simulink model "SSSC"  (R2022b)
settings: Solver=VariableStepAuto  StartTime=0.0  StopTime=.1  RelTol=1e-3
libraries: dspsigops x4, spsSeriesRLCBranchLib x3, simulink x2, spsDCVoltageSourceLib x2, spsMosfetLib x2, spsVoltageMeasurementLib x2, spsACVoltageSourceLib x1, spsCurrentMeasurementLib x1, spsTriangleGeneratorLib x1, sps_lib x1
settings Model: Creator=HP  LastModifiedBy=rishi kumar singh

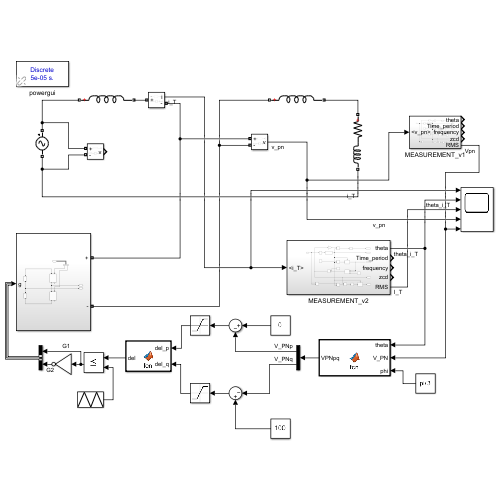
[thumbnail: Simulink's stored preview of the top-level diagram]
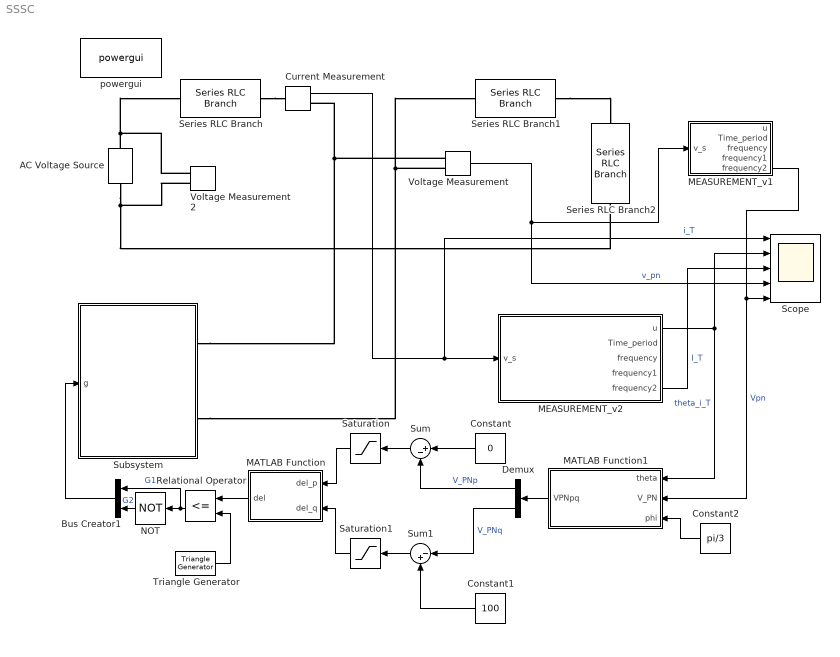
== system SSSC ==
  AC Voltage Source : spsACVoltageSourceLib/AC Voltage Source  Amplitude=20e3*sqrt(2)  Phase=0  Frequency=50  SampleTime=0  Measurements=None  BusType=swing  Pref=10e3  Qref=0  Qmin=-inf  Qmax=+inf
  Bus Creator1 : BusCreator  Inputs=2
  Constant : Constant  Value=0
  Constant1 : Constant  Value=100
  Constant2 : Constant  Value=pi/3
  Current Measurement : spsCurrentMeasurementLib/Current Measurement  PhasorSimulation=off  OutputType=Complex  PSBequivalent=0
  Demux : Demux  Outputs=2
  MATLAB Function : MATLAB Function  TreatAsAtomicUnit=on
  MATLAB Function1 : MATLAB Function  TreatAsAtomicUnit=on
  MEASUREMENT_v1 : Subsystem
  MEASUREMENT_v2 : Subsystem
  NOT : Logic  Operator=NOT  IconShape=distinctive  AllPortsSameDT=off  OutDataTypeStr=boolean
  Relational Operator : RelationalOperator  Operator=<=  OutDataTypeStr=boolean  RndMeth=Simplest  InputSameDT=off
  Saturation : Saturate
  Saturation1 : Saturate
  Scope : Scope  NumInputPorts=5
  Series RLC Branch : spsSeriesRLCBranchLib/Series RLC Branch  LConnTagsString=__new0  RConnTagsString=__new0  BranchType=L  Resistance=1  Inductance=5e-3  SetiL0=off  InitialCurrent=0  Capacitance=1e-6  Setx0=off  InitialVoltage=0  Measurements=None
  Series RLC Branch1 : spsSeriesRLCBranchLib/Series RLC Branch  LConnTagsString=__new0  RConnTagsString=__new0  BranchType=L  Resistance=1  Inductance=5e-3  SetiL0=off  InitialCurrent=0  Capacitance=1e-6  Setx0=off  InitialVoltage=0  Measurements=None
  Series RLC Branch2 : spsSeriesRLCBranchLib/Series RLC Branch  LConnTagsString=__new0  RConnTagsString=__new0  BranchType=RL  Resistance=10  Inductance=5e-3  SetiL0=off  InitialCurrent=0  Capacitance=1e-6  Setx0=off  InitialVoltage=0  Measurements=None
  Subsystem : Subsystem
  Sum : Sum  Inputs=|+-
  Sum1 : Sum  Inputs=|-+
  Triangle Generator : spsTriangleGeneratorLib/Triangle Generator  Freq=1e3  Phase=0  Ts=0
  Voltage Measurement : spsVoltageMeasurementLib/Voltage Measurement  PhasorSimulation=off  OutputType=Complex  PSBequivalent=0
  Voltage Measurement2 : spsVoltageMeasurementLib/Voltage Measurement  PhasorSimulation=off  OutputType=Complex  PSBequivalent=0
  powergui : sps_lib/powergui  Priority=1  SimulationMode=Discrete  SampleTime=50e-6  frequency=60  Iterations=50  frequencyindice=50  Pbase=100e6  ErrMax=1e-4  UnitsV=kV  UnitsW=MW  buscounter=0  FunctionMessages=off  echomessages=off  EnableUseOfTLC=off  CurrentSourceSwitches=off  DisableSnubberDevices=off  DisableRonSwitches=off  DisableVfSwitches=off  DisplayEquations=off  AutomaticDiscreteSolvers=off  SolverType=Tustin/Backward Euler (TBE)  Interpol=off  ExternalGateDelay=off  methode=off  Ts=100  x0status=blocks  SPID=on  SwTol=0  HookPort=off  NonlinearTolerance=1e-4  nMaxIteration=100  ContinueOnMaxIteration=off  RestoreLinks=warning  ResistiveCurrentMeasurement=off  Frange=[0:2:500]  Ylog=off  Xlog=on  ShowGrid=off  save=off  variable=ZData  structure=0  ZoomFFT=off  StartTime=0.0  cycles=1  DisplayStyle=1  fundamental=60  FreqAxis=off  MaxFrequency=1000  frequencyindicesteady=1  RmsSteady=1  display=off
  wires:
  MATLAB Function1/1(VPNpq) -> Demux/1
  MEASUREMENT_v2/1(u) -> Scope/2, MATLAB Function1/1(theta)  "theta_i_T"
  Bus Creator1/1 -> Subsystem/1(g)
  Current Measurement/1 -> Scope/1, MEASUREMENT_v2/1(v_s)  "i_T"
  MEASUREMENT_v2/5(frequency2) -> Scope/3  "I_T"
  Voltage Measurement/1 -> MEASUREMENT_v1/1(v_s), Scope/4  "v_pn"
  MEASUREMENT_v1/5(frequency2) -> MATLAB Function1/2(V_PN), Scope/5  "Vpn"
  Demux/1 -> Sum/2  "V_PNp"
  Demux/2 -> Sum1/1  "V_PNq"
  Sum/1 -> Saturation/1
  Sum1/1 -> Saturation1/1
  Constant/1 -> Sum/1
  Constant1/1 -> Sum1/2
  Saturation/1 -> MATLAB Function/1(del_p)
  Saturation1/1 -> MATLAB Function/2(del_q)
  MATLAB Function/1(del) -> Relational Operator/1
  Triangle Generator/1 -> Relational Operator/2
  NOT/1 -> Bus Creator1/2  "G2"
  Relational Operator/1 -> Bus Creator1/1, NOT/1  "G1"
  Constant2/1 -> MATLAB Function1/3(phi)
  connections:
  AC Voltage Source/RConn1 -- Voltage Measurement2/LConn1 -- Series RLC Branch/LConn1
  Series RLC Branch1/RConn1 -- Series RLC Branch2/LConn1
  Subsystem/RConn1 -- Voltage Measurement/LConn1 -- Current Measurement/RConn1
  AC Voltage Source/LConn1 -- Series RLC Branch2/RConn1 -- Voltage Measurement2/LConn2
  Subsystem/RConn2 -- Voltage Measurement/LConn2 -- Series RLC Branch1/LConn1
  Series RLC Branch/RConn1 -- Current Measurement/LConn1

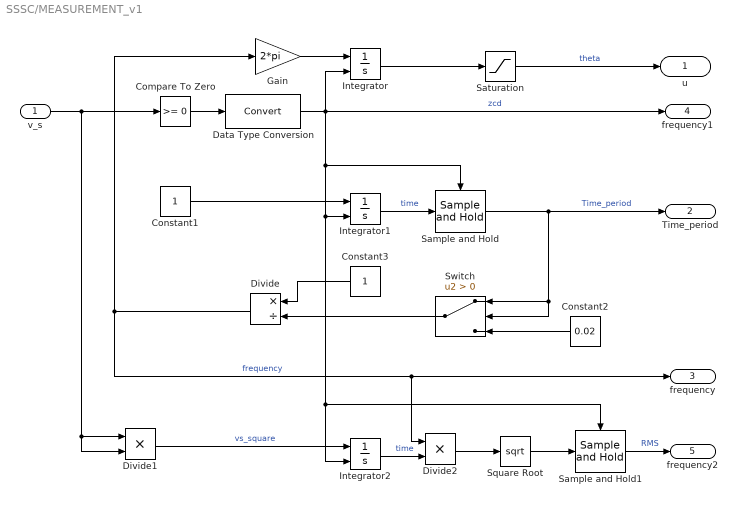
== system SSSC/MEASUREMENT_v1 ==
  v_s : Inport
  Compare To Zero : simulink/Logic and Bit Operations/Compare To Zero  relop=>=  OutDataTypeStr=boolean
  Constant1 : Constant
  Constant2 : Constant  Value=0.02
  Constant3 : Constant
  Data Type Conversion : DataTypeConversion  SaturateOnIntegerOverflow=off  RndMeth=Floor
  Divide : Product  Inputs=*/
  Divide1 : Product  Inputs=**
  Divide2 : Product  Inputs=**
  Gain : Gain  Gain=2*pi
  Integrator : Integrator  ExternalReset=rising
  Integrator1 : Integrator  ExternalReset=rising
  Integrator2 : Integrator  ExternalReset=rising
  Sample and Hold : dspsigops/Sample and Hold  trig=Rising edge  initCond=0  latchinput=on
  Sample and Hold1 : dspsigops/Sample and Hold  trig=Rising edge  initCond=0  latchinput=on
  Saturation : Saturate  UpperLimit=2*pi  LowerLimit=-2*pi
  Square Root : Sqrt
  Switch : Switch  Criteria=u2 > Threshold  SaturateOnIntegerOverflow=off  InputSameDT=off
  u : Outport
  Time_period : Outport  Port=2
  frequency : Outport  Port=3
  frequency1 : Outport  Port=4
  frequency2 : Outport  Port=5
  wires:
  Saturation/1 -> u/1  "theta"
  Sample and Hold1/1 -> frequency2/1  "RMS"
  Square Root/1 -> Sample and Hold1/1
  Divide2/1 -> Square Root/1
  Integrator2/1 -> Divide2/2  "time"
  Divide1/1 -> Integrator2/1  "vs_square"
  v_s/1 -> Compare To Zero/1, Divide1/1, Divide1/2
  Switch/1 -> Divide/2
  Integrator1/1 -> Sample and Hold/1  "time"
  Constant1/1 -> Integrator1/1
  Constant2/1 -> Switch/3
  Sample and Hold/1 -> Switch/1, Switch/2, Time_period/1  "Time_period"
  Gain/1 -> Integrator/1
  Data Type Conversion/1 -> Integrator/2, frequency1/1, Sample and Hold/Trigger, Integrator2/2, Sample and Hold1/Trigger, Integrator1/2  "zcd"
  Divide/1 -> frequency/1, Divide2/1, Gain/1  "frequency"
  Integrator/1 -> Saturation/1
  Constant3/1 -> Divide/1
  Compare To Zero/1 -> Data Type Conversion/1

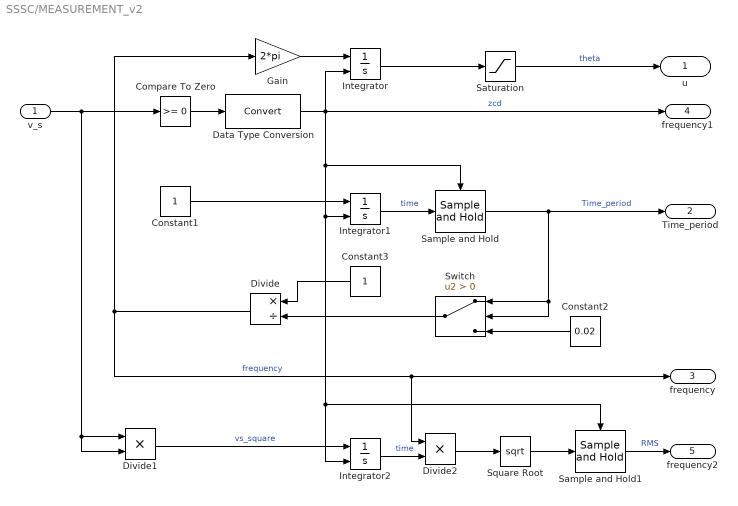
== system SSSC/MEASUREMENT_v2 ==
  v_s : Inport
  Compare To Zero : simulink/Logic and Bit Operations/Compare To Zero  relop=>=  OutDataTypeStr=boolean
  Constant1 : Constant
  Constant2 : Constant  Value=0.02
  Constant3 : Constant
  Data Type Conversion : DataTypeConversion  SaturateOnIntegerOverflow=off  RndMeth=Floor
  Divide : Product  Inputs=*/
  Divide1 : Product  Inputs=**
  Divide2 : Product  Inputs=**
  Gain : Gain  Gain=2*pi
  Integrator : Integrator  ExternalReset=rising
  Integrator1 : Integrator  ExternalReset=rising
  Integrator2 : Integrator  ExternalReset=rising
  Sample and Hold : dspsigops/Sample and Hold  trig=Rising edge  initCond=0  latchinput=on
  Sample and Hold1 : dspsigops/Sample and Hold  trig=Rising edge  initCond=0  latchinput=on
  Saturation : Saturate  UpperLimit=2*pi  LowerLimit=-2*pi
  Square Root : Sqrt
  Switch : Switch  Criteria=u2 > Threshold  SaturateOnIntegerOverflow=off  InputSameDT=off
  u : Outport
  Time_period : Outport  Port=2
  frequency : Outport  Port=3
  frequency1 : Outport  Port=4
  frequency2 : Outport  Port=5
  wires:
  Compare To Zero/1 -> Data Type Conversion/1
  Constant3/1 -> Divide/1
  Integrator/1 -> Saturation/1
  Divide/1 -> Gain/1, Divide2/1, frequency/1  "frequency"
  Data Type Conversion/1 -> Integrator1/2, Sample and Hold1/Trigger, Integrator2/2, Sample and Hold/Trigger, frequency1/1, Integrator/2  "zcd"
  Gain/1 -> Integrator/1
  Sample and Hold/1 -> Time_period/1, Switch/2, Switch/1  "Time_period"
  Constant2/1 -> Switch/3
  Constant1/1 -> Integrator1/1
  Integrator1/1 -> Sample and Hold/1  "time"
  Switch/1 -> Divide/2
  v_s/1 -> Divide1/2, Divide1/1, Compare To Zero/1
  Divide1/1 -> Integrator2/1  "vs_square"
  Integrator2/1 -> Divide2/2  "time"
  Divide2/1 -> Square Root/1
  Square Root/1 -> Sample and Hold1/1
  Sample and Hold1/1 -> frequency2/1  "RMS"
  Saturation/1 -> u/1  "theta"

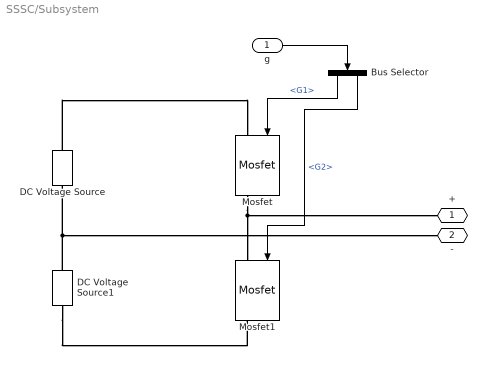
== system SSSC/Subsystem ==
  g : Inport
  Bus Selector : BusSelector  OutputSignals=G1,G2
  DC Voltage Source : spsDCVoltageSourceLib/DC Voltage Source  Amplitude=(20e3)*sqrt(2)/2  Measurements=None
  DC Voltage Source1 : spsDCVoltageSourceLib/DC Voltage Source  Amplitude=(20e3)*sqrt(2)/2  Measurements=None
  Mosfet : spsMosfetLib/Mosfet  Ron=0.1  Lon=0  Rd=0.01  Vfd=0  IC=0  Rs=1e5  Cs=inf  Measurements=on
  Mosfet1 : spsMosfetLib/Mosfet  Ron=0.1  Lon=0  Rd=0.01  Vfd=0  IC=0  Rs=1e5  Cs=inf  Measurements=on
  + : PMIOPort  Side=Right
  - : PMIOPort  Port=2  Side=Right
  wires:
  Bus Selector/1 -> Mosfet/1  "<G1>"
  Bus Selector/2 -> Mosfet1/1  "<G2>"
  g/1 -> Bus Selector/1
  connections:
  Mosfet/RConn1 -- Mosfet1/LConn1 -- +/RConn1
  DC Voltage Source/RConn1 -- Mosfet/LConn1
  DC Voltage Source1/RConn1 -- DC Voltage Source/LConn1 -- -/RConn1
  DC Voltage Source1/LConn1 -- Mosfet1/RConn1

== matlab function SSSC/MATLAB Function1 ==
  data: theta input; VPNpq output; V_PN input; phi input
function VPNpq = fcn(theta, V_PN, phi)
VPNpq = [0 0];
V_PNpf = V_PN*cos(phi);
V_PNqf = V_PN*sin(phi);
if (theta>= 0 && theta < pi)
V_PNpq = [V_PNpf V_PNqf];
end

if (theta>= pi && theta < 2*pi)
V_PNpq = [V_PNpf V_PNqf];
end

== matlab function SSSC/MATLAB Function ==
  data: del_p input; del output; del_q input
function del = fcn(del_p,del_q)
del = sqrt(del_p^2 + del_q^2);
del ;
